simulink model "c8mblk2"  (R2019b)
settings: Solver=ode45  StartTime=0.0  StopTime=10  RelTol=1e-7  EnableMultiTasking=on
PreLoadFcn:
  |  ww=[1e-5 1e5]; N=20;
libraries: cstblocks x6
settings Model: Creator=Dingyu  LastModifiedBy=xuedi
settings DataIOCC: SaveFormat=Array  ReturnWorkspaceOutputs=off
settings OptimizationCC: LifeSpan=inf
settings DebuggingCC: AllowSymbolicDim=off  SFUnexpectedBacktrackingDiag=warning  SFNoUnconditionalDefaultTransitionDiag=warning  ArithmeticOperatorsInVariantConditions=warning
settings ModelReferenceCC: PropagateSignalLabelsOutOfModel=off
settings SFSimCC: SimUseLocalCustomCode=off  CustomCodeUndefinedFunction=UseInterfaceOnly
settings RTWCC: RTWUseLocalCustomCode=off
settings CodeAppCC: StateflowObjectComments=on
settings GRTTargetCC: TargetLangStandard=C89/C90 (ANSI)
settings ConfigComp: CovMetricSettings=dw  CovSaveCumulativeToWorkspaceVar=on  CovSaveSingleToWorkspaceVar=on  CovExternalEMLEnable=off

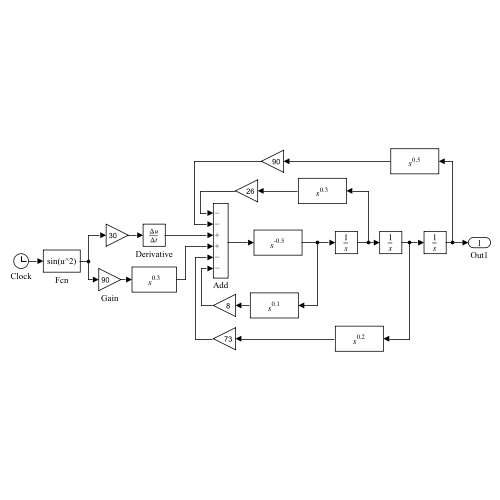
[thumbnail: Simulink's stored preview of the top-level diagram]
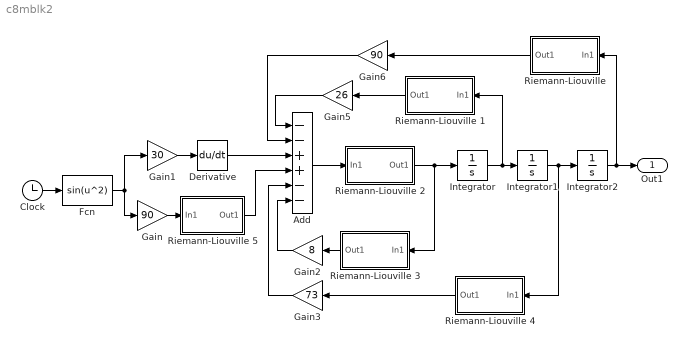
== system c8mblk2 ==
  Add : Sum  Inputs=--++--
  Clock : Clock
  Derivative : Derivative
  Fcn : Fcn  Expr=sin(u^2)
  Gain : Gain  Gain=90
  Gain1 : Gain  Gain=30
  Gain2 : Gain  Gain=8
  Gain3 : Gain  Gain=73
  Gain5 : Gain  Gain=26
  Gain6 : Gain  Gain=90
  Integrator : Integrator
  Integrator1 : Integrator
  Integrator2 : Integrator
  "Riemann-Liouville " : Subsystem  mask{gam=0.5, ww=ww, n=N, kF1=on, kF=Oustaloup filter}
      mask prompts: gam "Derivative order gamma"; ww "Frequency range [wb,wh]"; n "Apprixmation order"; kF1 "Is a low-pass filter required?"; kF "Filter type"
      mask init:
      | wb=ww(1); wh=ww(2); 
      | if isnumeric(gam), str=['{\its}^{' num2str(gam) '}']; 
      | else, str='{\its}^{\gamma}'; end
      | if kF==1, G=ousta_fod(gam,n,wb,wh);
      | elseif kF==2, G=new_fod(gam,n,wb,wh); 
      | else, G=matsuda_fod(gam,n,wb,wh); end
      | T=1/wh; if kF1==1, G=G*tf(1,[T 1]); end
      mask TypeOptions kF: Oustaloup filter | Modified Oustaloup filter | Matsuda-Fujii filter
      mask Display: disp(str,'texmode','on')
  Riemann-Liouville 1 : Subsystem  mask{gam=0.3, ww=ww, n=N, kF1=on, kF=Oustaloup filter}
      mask prompts: gam "Derivative order gamma"; ww "Frequency range [wb,wh]"; n "Apprixmation order"; kF1 "Is a low-pass filter required?"; kF "Filter type"
      mask init: same as c8mblk2/Riemann-Liouville 
      mask TypeOptions kF: Oustaloup filter | Modified Oustaloup filter | Matsuda-Fujii filter
      mask Display: disp(str,'texmode','on')
  Riemann-Liouville 2 : Subsystem  mask{gam=-0.5, ww=ww, n=N, kF1=on, kF=Oustaloup filter}
      mask prompts: gam "Derivative order gamma"; ww "Frequency range [wb,wh]"; n "Apprixmation order"; kF1 "Is a low-pass filter required?"; kF "Filter type"
      mask init: same as c8mblk2/Riemann-Liouville 
      mask TypeOptions kF: Oustaloup filter | Modified Oustaloup filter | Matsuda-Fujii filter
      mask Display: disp(str,'texmode','on')
  Riemann-Liouville 3 : Subsystem  mask{gam=0.1, ww=ww, n=N, kF1=on, kF=Oustaloup filter}
      mask prompts: gam "Derivative order gamma"; ww "Frequency range [wb,wh]"; n "Apprixmation order"; kF1 "Is a low-pass filter required?"; kF "Filter type"
      mask init: same as c8mblk2/Riemann-Liouville 
      mask TypeOptions kF: Oustaloup filter | Modified Oustaloup filter | Matsuda-Fujii filter
      mask Display: disp(str,'texmode','on')
  Riemann-Liouville 4 : Subsystem  mask{gam=0.2, ww=ww, n=N, kF1=on, kF=Oustaloup filter}
      mask prompts: gam "Derivative order gamma"; ww "Frequency range [wb,wh]"; n "Apprixmation order"; kF1 "Is a low-pass filter required?"; kF "Filter type"
      mask init: same as c8mblk2/Riemann-Liouville 
      mask TypeOptions kF: Oustaloup filter | Modified Oustaloup filter | Matsuda-Fujii filter
      mask Display: disp(str,'texmode','on')
  Riemann-Liouville 5 : Subsystem  mask{gam=0.3, ww=ww, n=N, kF1=on, kF=Oustaloup filter}
      mask prompts: gam "Derivative order gamma"; ww "Frequency range [wb,wh]"; n "Apprixmation order"; kF1 "Is a low-pass filter required?"; kF "Filter type"
      mask init: same as c8mblk2/Riemann-Liouville 
      mask TypeOptions kF: Oustaloup filter | Modified Oustaloup filter | Matsuda-Fujii filter
      mask Display: disp(str,'texmode','on')
  Out1 : Outport
  wires:
  Integrator/1 -> Riemann-Liouville 1/1(In1), Integrator1/1
  Riemann-Liouville 2/1(Out1) -> Riemann-Liouville 3/1(In1), Integrator/1
  Integrator1/1 -> Riemann-Liouville 4/1(In1), Integrator2/1
  Derivative/1 -> Add/3
  Gain/1 -> Riemann-Liouville 5/1(In1)
  Clock/1 -> Fcn/1
  Fcn/1 -> Gain/1, Gain1/1
  Gain1/1 -> Derivative/1
  Gain2/1 -> Add/6
  Gain3/1 -> Add/5
  Integrator2/1 -> "Riemann-Liouville "/1(In1), Out1/1
  Gain5/1 -> Add/1
  Gain6/1 -> Add/2
  Add/1 -> Riemann-Liouville 2/1(In1)
  "Riemann-Liouville "/1(Out1) -> Gain6/1
  Riemann-Liouville 1/1(Out1) -> Gain5/1
  Riemann-Liouville 3/1(Out1) -> Gain2/1
  Riemann-Liouville 4/1(Out1) -> Gain3/1
  Riemann-Liouville 5/1(Out1) -> Add/4

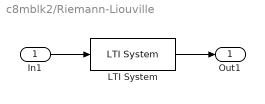
== system c8mblk2/Riemann-Liouville  ==
  In1 : Inport
  LTI System : cstblocks/LTI System  sys=G  IC=[]
  Out1 : Outport
  wires:
  In1/1 -> LTI System/1
  LTI System/1 -> Out1/1

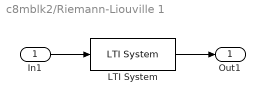
== system c8mblk2/Riemann-Liouville 1 ==
  In1 : Inport
  LTI System : cstblocks/LTI System  sys=G  IC=[]
  Out1 : Outport
  wires:
  LTI System/1 -> Out1/1
  In1/1 -> LTI System/1

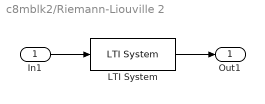
== system c8mblk2/Riemann-Liouville 2 ==
  In1 : Inport
  LTI System : cstblocks/LTI System  sys=G  IC=[]
  Out1 : Outport
  wires:
  In1/1 -> LTI System/1
  LTI System/1 -> Out1/1

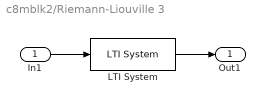
== system c8mblk2/Riemann-Liouville 3 ==
  In1 : Inport
  LTI System : cstblocks/LTI System  sys=G  IC=[]
  Out1 : Outport
  wires:
  LTI System/1 -> Out1/1
  In1/1 -> LTI System/1

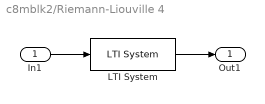
== system c8mblk2/Riemann-Liouville 4 ==
  In1 : Inport
  LTI System : cstblocks/LTI System  sys=G  IC=[]
  Out1 : Outport
  wires:
  In1/1 -> LTI System/1
  LTI System/1 -> Out1/1

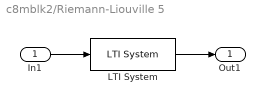
== system c8mblk2/Riemann-Liouville 5 ==
  In1 : Inport
  LTI System : cstblocks/LTI System  sys=G  IC=[]
  Out1 : Outport
  wires:
  LTI System/1 -> Out1/1
  In1/1 -> LTI System/1
